simulink model "Simulation_Nonlinear_MRAC_v2"  (R2023b)
settings: Solver=VariableStepAuto  StartTime=0.0  StopTime=Tsim  RelTol=1e-3
undefined symbols (not defined in the file): a, am, amplitude, b, BETA, BETA_m, bias, bm, epsilon, IC_P, IC_Pm, period, phase_delay, pulse_width, SAT_ACTIVE, SIGNAL_NR, w, WEIGHT_UPDATE, wm
settings Model: Creator=dalimwahby  LastModifiedBy=dalimwahby

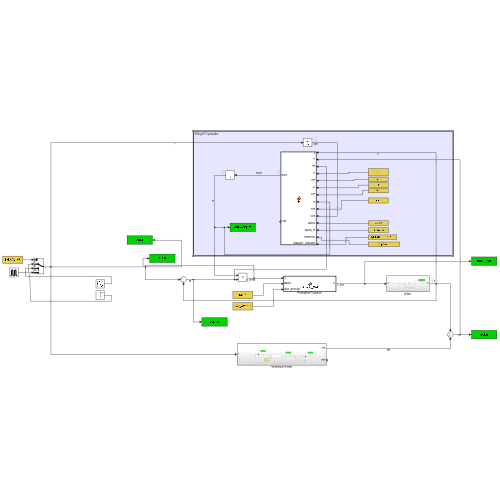
[thumbnail: Simulink's stored preview of the top-level diagram]
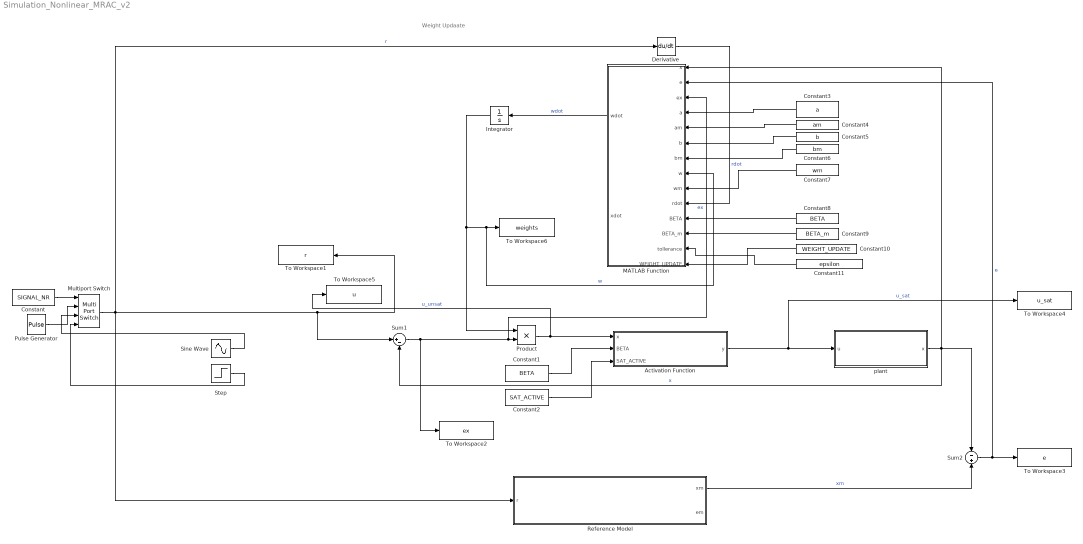
== system Simulation_Nonlinear_MRAC_v2 ==
  note: Weight Updaate
  Activation Function : MATLAB Function  TreatAsAtomicUnit=on
  Constant : Constant  Value=SIGNAL_NR
  Constant1 : Constant  Value=BETA
  Constant10 : Constant  Value=WEIGHT_UPDATE
  Constant11 : Constant  Value=epsilon
  Constant2 : Constant  Value=SAT_ACTIVE
  Constant3 : Constant  Value=a
  Constant4 : Constant  Value=am
  Constant5 : Constant  Value=b
  Constant6 : Constant  Value=bm
  Constant7 : Constant  Value=wm
  Constant8 : Constant  Value=BETA
  Constant9 : Constant  Value=BETA_m
  Derivative : Derivative
  Integrator : Integrator  InitialCondition=w
  MATLAB Function : MATLAB Function  TreatAsAtomicUnit=on
  Multiport Switch : MultiPortSwitch  SaturateOnIntegerOverflow=off  InputSameDT=off
  Product : Product
  Pulse Generator : DiscretePulseGenerator  PulseType=Time based  Amplitude=amplitude  Period=period  PulseWidth=pulse_width*100  PhaseDelay=phase_delay
  Reference Model : Subsystem
  Sine Wave : Sin  Amplitude=amplitude  Bias=bias  SampleTime=0
  Step : Step  Time=phase_delay  After=amplitude  SampleTime=0
  Sum1 : Sum  Inputs=|+-
  Sum2 : Sum  Inputs=-+
  To Workspace1 : ToWorkspace  VariableName=r  SaveFormat=Timeseries  SampleTime=-1
  To Workspace2 : ToWorkspace  VariableName=ex  SaveFormat=Timeseries  SampleTime=-1
  To Workspace3 : ToWorkspace  VariableName=e  SaveFormat=Timeseries  SampleTime=-1
  To Workspace4 : ToWorkspace  VariableName=u_sat  SaveFormat=Timeseries  SampleTime=-1
  To Workspace5 : ToWorkspace  VariableName=u  SaveFormat=Timeseries  SampleTime=-1
  To Workspace6 : ToWorkspace  VariableName=weights  SaveFormat=Timeseries  SampleTime=-1
  plant : Subsystem
  wires:
  plant/1(x) -> Sum2/1, Sum1/2, MATLAB Function/1(x)  "x"
  Constant1/1 -> Activation Function/2(BETA)
  Multiport Switch/1 -> To Workspace1/1, Sum1/1, Derivative/1, Reference Model/1(r)  "r"
  Step/1 -> Multiport Switch/4
  Activation Function/1(y) -> plant/1(u), To Workspace4/1  "u_sat"
  Sum1/1 -> MATLAB Function/3(ex), Product/2, To Workspace2/1  "ex"
  Reference Model/1(xm) -> Sum2/2  "xm"
  Sum2/1 -> MATLAB Function/2(e), To Workspace3/1  "e"
  Constant2/1 -> Activation Function/3(SAT_ACTIVE)
  Product/1 -> To Workspace5/1, Activation Function/1(x)  "u_unsat"
  Constant/1 -> Multiport Switch/1
  Sine Wave/1 -> Multiport Switch/3
  Pulse Generator/1 -> Multiport Switch/2
  MATLAB Function/1(wdot) -> Integrator/1  "wdot"
  Constant3/1 -> MATLAB Function/4(a)
  Constant5/1 -> MATLAB Function/6(b)
  Constant11/1 -> MATLAB Function/13(tollerance)
  Constant7/1 -> MATLAB Function/9(wm)
  Integrator/1 -> MATLAB Function/8(w), To Workspace6/1, Product/1  "w"
  Constant4/1 -> MATLAB Function/5(am)
  Constant10/1 -> MATLAB Function/14(WEIGHT_UPDATE)
  Constant9/1 -> MATLAB Function/12(BETA_m)
  Constant6/1 -> MATLAB Function/7(bm)
  Constant8/1 -> MATLAB Function/11(BETA)
  Derivative/1 -> MATLAB Function/10(rdot)  "rdot"

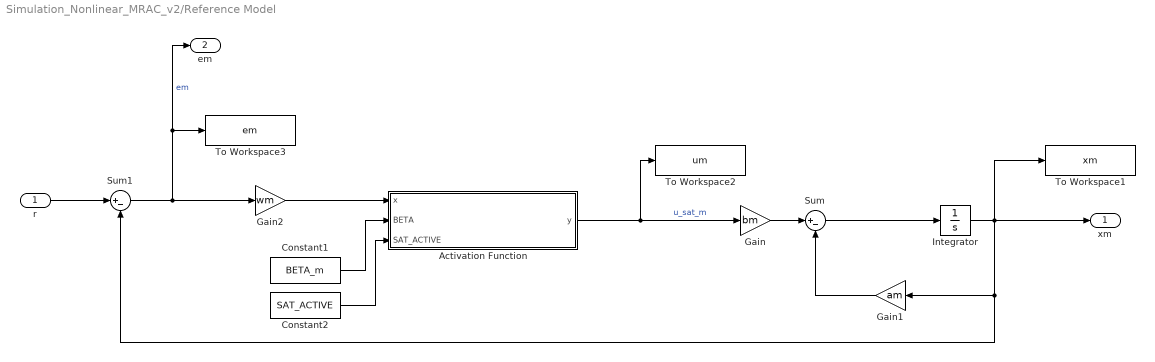
== system Simulation_Nonlinear_MRAC_v2/Reference Model ==
  r : Inport
  Activation Function : MATLAB Function  TreatAsAtomicUnit=on
  Constant1 : Constant  Value=BETA_m
  Constant2 : Constant  Value=SAT_ACTIVE
  Gain : Gain  Gain=bm
  Gain1 : Gain  Gain=am
  Gain2 : Gain  Gain=wm
  Integrator : Integrator  InitialCondition=IC_Pm
  Sum : Sum  Inputs=|+-
  Sum1 : Sum  Inputs=|+-
  To Workspace1 : ToWorkspace  VariableName=xm  SaveFormat=Timeseries  SampleTime=-1
  To Workspace2 : ToWorkspace  VariableName=um  SaveFormat=Timeseries  SampleTime=-1
  To Workspace3 : ToWorkspace  VariableName=em  SaveFormat=Timeseries  SampleTime=-1
  xm : Outport
  em : Outport  Port=2
  wires:
  Constant2/1 -> Activation Function/3(SAT_ACTIVE)
  Sum/1 -> Integrator/1
  Constant1/1 -> Activation Function/2(BETA)
  Gain1/1 -> Sum/2
  Activation Function/1(y) -> To Workspace2/1, Gain/1  "u_sat_m"
  Integrator/1 -> Sum1/2, Gain1/1, xm/1, To Workspace1/1
  Gain/1 -> Sum/1
  Gain2/1 -> Activation Function/1(x)
  r/1 -> Sum1/1
  Sum1/1 -> em/1, To Workspace3/1, Gain2/1  "em"

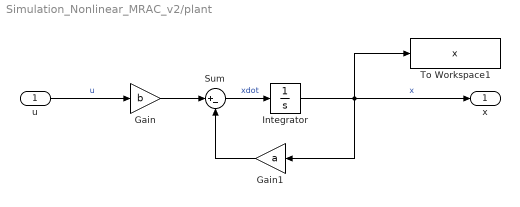
== system Simulation_Nonlinear_MRAC_v2/plant ==
  u : Inport
  Gain : Gain  Gain=b
  Gain1 : Gain  Gain=a
  Integrator : Integrator  InitialCondition=IC_P
  Sum : Sum  Inputs=|+-
  To Workspace1 : ToWorkspace  VariableName=x  SaveFormat=Timeseries  SampleTime=-1
  x : Outport
  wires:
  u/1 -> Gain/1  "u"
  Sum/1 -> Integrator/1  "xdot"
  Integrator/1 -> Gain1/1, x/1, To Workspace1/1  "x"
  Gain1/1 -> Sum/2
  Gain/1 -> Sum/1

== matlab function Simulation_Nonlinear_MRAC_v2/Activation Function ==
  data: x input; y output; BETA input; SAT_ACTIVE input
function y = Sigmoid_SAT(x, BETA, SAT_ACTIVE)
    if SAT_ACTIVE==1
        y = (2*(1-exp(-BETA.*x)))./(BETA*(1+exp(-BETA.*x)));
    else
        y = x;
    end
end

== matlab function Simulation_Nonlinear_MRAC_v2/Reference Model/Activation Function ==
  data: x input; y output; BETA input; SAT_ACTIVE input
function y = Sigmoid_SAT(x, BETA, SAT_ACTIVE)
    if SAT_ACTIVE==1
        y = (2*(1-exp(-BETA.*x)))./(BETA*(1+exp(-BETA.*x)));
    else
        y = x;
    end
end

== matlab function Simulation_Nonlinear_MRAC_v2/MATLAB Function ==
  data: x input; e input; wdot output; ex input; a input; am input; b input; bm input; w input; wm input; rdot input; BETA input; BETA_m input; tollerance input; WEIGHT_UPDATE input; xdot output
function [wdot, xdot] = fcn(x, e, ex, a, am, b ,bm, w, wm, rdot, BETA, BETA_m, tollerance, WEIGHT_UPDATE)
if WEIGHT_UPDATE==1
    %% If ex is equal to zero, do not update the weights due to zero division
    if abs(ex)<=tollerance
        wdot=0;

        input_ex = w*ex;
        sigma_ex = (2*(1-exp(-BETA.*input_ex)))./(BETA*(1+exp(-BETA.*input_ex)));

        xdot = -a*x+b*sigma_ex;

    else
        %% System
        input_ex = w*ex;
        sigma_ex = (2*(1-exp(-BETA.*input_ex)))./(BETA*(1+exp(-BETA.*input_ex)));
        
        xdot = -a*x+b*sigma_ex;
        
        exdot = rdot-xdot;
    
        dsigma_ex = (4*exp(-BETA.*input_ex))./((1+exp(-BETA.*input_ex)).^2);
        
        %% Model reference
        input_em = wm*ex;
        %sigma_em = (2*(1-exp(-BETA_m.*input_em)))./(BETA_m*(1+exp(-BETA_m.*input_em)));

        %xmdot = -am*xm+bm*sigma_em;
        
        %emdot = rdot-xmdot;
        emdot=exdot;
    
        dsigma_em = (4*exp(-BETA_m.*input_em))./((1+exp(-BETA_m.*input_em)).^2);
    
    
        %% Time derivative of weights
        wdot = ((1/(ex*b*dsigma_ex))*(e + (a-am)*xdot + bm*dsigma_em*wm*emdot)-((w/ex)*exdot));

    end
else
    wdot=0;

    input_ex = w*ex;
    sigma_ex = (2*(1-exp(-BETA.*input_ex)))./(BETA*(1+exp(-BETA.*input_ex)));

    xdot = -a*x+b*sigma_ex;
end
